simulink model "Tricopter_Controlled"  (R2015a)
settings: Solver=ode3  SolverMode=SingleTasking  StartTime=0.0  StopTime=inf  FixedStep=T_sim  RelTol=1e-3
values from neighbouring files (symbols this model uses):
  A_l_max_x = sqrt( (A_z_max)^2  -  g^2  )    [Run3Copter.m]
  A_l_max_y = g*tand(15)    [Run3Copter.m]
  A_z_max = Max_Thrust*3/m    [Run3Copter.m]
  Alt_0 = input(' Give the initial altitude (m): ')    [Run3Copter.m]
  B_hover_4dof = [-0.192641491537 -0.295051706147 -72.3190840892 -0.00308714144823 24.9504828653 -1.18743631629 9.87469464114e-05 6.48783896558 -0.0529805907426 -0.000387203135788 0.131620058452 2.24065603044 ... (54 elements, 6x9)]    [Effectiv_matrices.mat]
  CG_0 = [0,0,0.02]'    [SetupComplete.m]
  epsilon = 0.01    [Run3Copter.m]
  eta_23 = deg2rad(-1.3)    [Run3Copter.m]
  g = 9.81    [SetupComplete.m]
  h = 0.08    [SetupComplete.m]
  h_M = 0.064    [SetupComplete.m]
  Hover_eta_23 = deg2rad(-1.3)    [Run3Copter.m]
  Hover_throtle_1 = 0.745    [Run3Copter.m]
  Hover_throtle_23 = Hover_throtle_1/cos(Hover_eta_23)    [Run3Copter.m]
  I_BAC_0 = [ Ix,0,Ixz;0,Iy,0;Ixz,0,Iz]    [SetupComplete.m]
  Initial_Omegas = Omega_hover    [Run3Copter.m]
  Initial_Torques = Torque_hover    [Run3Copter.m]
  Ix = 0.103    [SetupComplete.m]
  Iy = 0.147    [SetupComplete.m]
  Iz = 0.237    [SetupComplete.m]
  l = 0.345    [SetupComplete.m]
  l_arm = 0.264    [SetupComplete.m]
  latitude = 52.071118    [Run3Copter.m]
  longitude = -0.627404    [Run3Copter.m]
  m = 3.51    [SetupComplete.m]
  m_0 = 2.61    [SetupComplete.m]
  m_M = 0.300    (= 0.3)    [SetupComplete.m]
  Rotation_sign = [ 1,-1,-1]    [SetupComplete.m]
  T_ctrl = 0.02    [Run3Copter.m]
  T_sim = 0.01    [Run3Copter.m]
  throtle_1 = 0*0.745    (= 0)    [Run3Copter.m]
  throtle_23 = throtle_1/cos(eta_23)    [Run3Copter.m]
  v_i0 = sqrt( 1/3*m*g/(2*rho*pi*R^2)  )    [SetupComplete.m]
undefined symbols (not defined in the file or in its folder): DOWN_0, EAST_0, Newton, NORTH_0, P_0, Q_0, R_0, Raphson, U_0, V_0, W_0
libraries: XXCopter_Control x64, simulink_extras x17, simulink x11, XXCopter x8
(part 1 of 6)
settings Model: ExtModeTrigDuration=5000  Creator=DavidTorres  LastModifiedBy=David
settings SolverCC: AutoInsertRateTranBlk=on
settings DataIOCC: LimitDataPoints=off  SaveOutput=off  SignalLogging=off  DSMLogging=off  VisualizeSimOutput=off  SaveTime=off
settings OptimizationCC: InlineParams=on  UseFloatMulNetSlope=on  UseSpecifiedMinMax=on  InlineInvariantSignals=on  EnhancedBackFolding=on  PassReuseOutputArgsAs=Individual arguments  ZeroExternalMemoryAtStartup=off  ZeroInternalMemoryAtStartup=off  EfficientFloat2IntCast=on  EfficientMapNaN2IntZero=off  OptimizeModelRefInitCode=on  LifeSpan=Inf  MaxStackSize=inf
settings DebuggingCC: WriteAfterWriteMsg=EnableAllAsError  SaveWithParameterizedLinksMsg=none  SignalResolutionControl=TryResolveAllWithWarning  IntegerOverflowMsg=error  ParameterUnderflowMsg=error  ParameterTunabilityLossMsg=error  UniqueDataStoreMsg=error  StrictBusMsg=ErrorOnBusTreatedAsVector  NonBusSignalsTreatedAsBus=error  SFUnexpectedBacktrackingDiag=error  SFInvalidInputDataAccessInChartInitDiag=error  SFNoUnconditionalDefaultTransitionDiag=error  SFTransitionOutsideNaturalParentDiag=error  SFUnconditionalTransitionShadowingDiag=error  SFUndirectedBroadcastEventsDiag=error  SFTransitionActionBeforeConditionDiag=error  IntegerSaturationMsg=error
settings HardwareCC: ProdLargestAtomicInteger=Long  ProdLargestAtomicFloat=Float  ProdIntDivRoundTo=Zero  ProdEndianess=LittleEndian  ProdHWDeviceType=ARM Compatible->ARM 10
settings RTWCC: SystemTargetFile=ert.tlc  GenCodeOnly=on  TemplateMakefile=ert_default_tmf  Description=Embedded Coder  BuildConfiguration=Faster Runs  CheckMdlBeforeBuild=Warning
settings CodeAppCC: IgnoreCustomStorageClasses=off  IgnoreTestpoints=on
settings ERTTargetCC: UtilityFuncGeneration=Shared location  ParMdlRefBuildCompliant=on  CompOptLevelCompliant=on  ConcurrentExecutionCompliant=on  IncludeMdlTerminateFcn=off  ERTFirstTimeCompliant=on  SupportAbsoluteTime=off  SupportNonFinite=off  SupportContinuousTime=off  ParenthesesLevel=Minimum  ModelStepFunctionPrototypeControlCompliant=on  CPPClassGenCompliant=on  ERTCustomFileTemplate=example_file_process.tlc  PreserveIfCondition=on  ConvertIfToSwitch=on

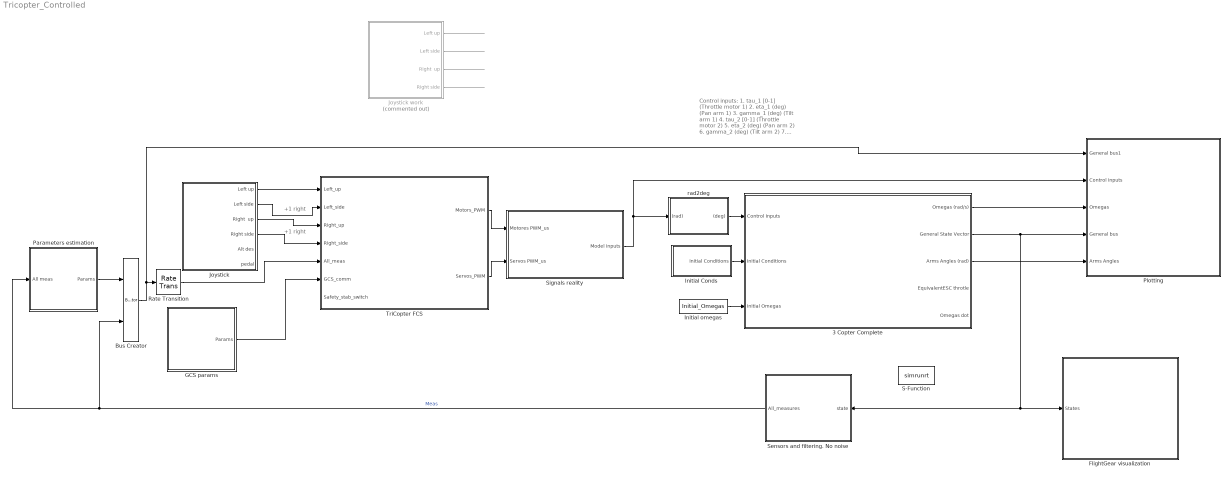
== system Tricopter_Controlled ==
  note: +1 right
  note: Control inputs:
      | 1. tau_1 [0-1] (Throttle motor 1)
      | 2. eta_1 (deg)  (Pan arm 1)
      | 3. gamma_1 (deg)  (Tilt arm 1)
      |
      | 4. tau_2 [0-1] (Throttle motor 2)
      | 5. eta_2 (deg)  (Pan arm 2)
      | 6. gamma_2 (deg)  (Tilt arm 2)
      |
      | 7. tau_3 [0-1] (Throttle motor 3)
      | 8. eta_3 (deg)  (Pan arm  3)
      | 9. gamma_3 (deg)  (Tilt arm 3)
  note: +1 right
  3 Copter Complete : Subsystem
  Bus Creator : BusCreator  Inputs=2
  FlightGear visualization : Subsystem
      mask Display:
      | % disp('{\bf\fontsize{20} Flight Gear}', 'texmode','on');
      | % image('FG F16.jpg')
      | % image(imread('FlightGear_logo.png'))
  GCS params : Subsystem  TreatAsAtomicUnit=on
  Initial Conds : Subsystem  TreatAsAtomicUnit=on
  Initial omegas : Constant  Value=Initial_Omegas
  Joystick : Subsystem
  Joystick work : Subsystem  Commented=on
  Parameters estimation : Subsystem  TreatAsAtomicUnit=on
  Plotting : Subsystem  SystemSampleTime=T_ctrl
  Rate Transition : RateTransition  OutPortSampleTime=T_ctrl
  S-Function : S-Function  FunctionName=simrunrt  Parameters=1
  Sensors and filtering. No noise : Subsystem  Variant=on  VariantControl=No noise  OverrideUsingVariant=No noise
  Signals reality : Subsystem
  TriCopter FCS : Subsystem
  rad2deg : Subsystem  TreatAsAtomicUnit=on
  wires:
  Initial omegas/1 -> 3 Copter Complete/3(Initial Omegas)
  Initial Conds/1(Initial Conditions) -> 3 Copter Complete/2(Initial Conditions)
  3 Copter Complete/1(Omegas (rad/s)) -> Plotting/3(Omegas)
  3 Copter Complete/3(Arms Angles (rad)) -> Plotting/5(Arms Angles)
  rad2deg/1((deg)) -> 3 Copter Complete/1(Control Inputs)
  Sensors and filtering. No noise/1(All_measures) -> Parameters estimation/1(All meas), Bus Creator/2  "Meas"
  3 Copter Complete/2(General State Vector) -> Plotting/4(General bus), Sensors and filtering. No noise/1(state), FlightGear visualization/1(States)
  Bus Creator/1 -> Rate Transition/1, Plotting/1(General bus1)
  Parameters estimation/1(Params) -> Bus Creator/1
  Signals reality/1(Model inputs) -> Plotting/2(Control inputs), rad2deg/1((rad))
  TriCopter FCS/1(Motors_PWM) -> Signals reality/1(Motores PWM_us)
  TriCopter FCS/2(Servos_PWM) -> Signals reality/2(Servos PWM_us)
  GCS params/1(Params) -> TriCopter FCS/6(GCS_comm)
  Joystick/1(Left up) -> TriCopter FCS/1(Left_up)
  Joystick/2(Left side) -> TriCopter FCS/2(Left_side)
  Joystick/3(Right  up) -> TriCopter FCS/3(Right_up)
  Joystick/4(Right side) -> TriCopter FCS/4(Right_side)
  Joystick work/4(Right side) -> ?
  Joystick work/1(Left up) -> ?
  Joystick work/2(Left side) -> ?
  Joystick work/3(Right  up) -> ?
  Rate Transition/1 -> TriCopter FCS/5(All_meas)

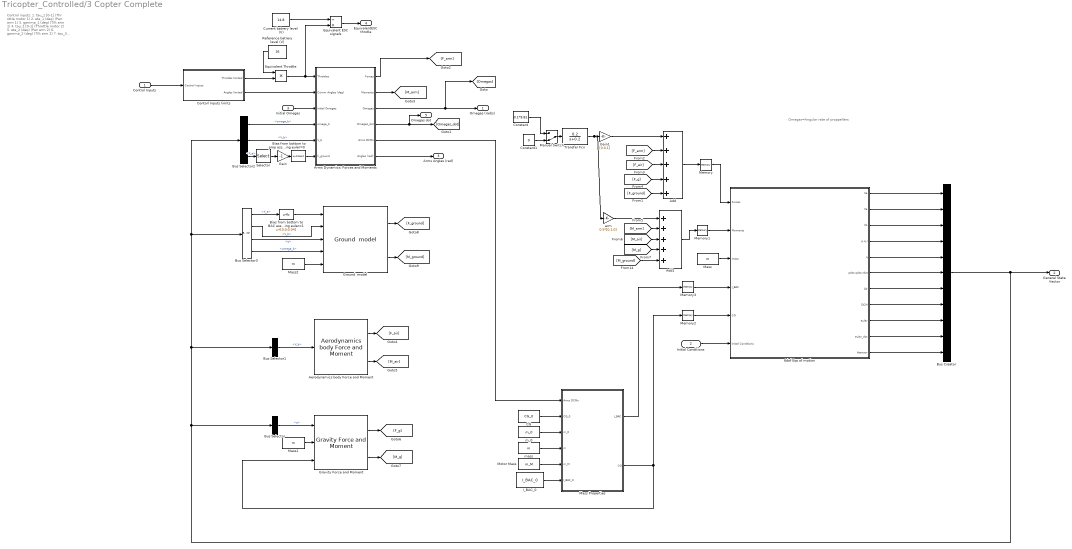
== system Tricopter_Controlled/3 Copter Complete ==
  note: Omegas=Angular rate of proppellers
  note: Control inputs:
      | 1. tau_1 [0-1] (Thr ottle motor 1)
      | 2. eta_1 (deg)  (Pan arm 1)
      | 3. gamma_1 (deg)  (Tilt arm 1)
      |
      | 4. tau_2 [0-1] (Throttle motor 2)
      | 5. eta_2 (deg)  (Pan arm 2)
      | 6. gamma_2 (deg)  (Tilt arm 2)
      |
      | 7. tau_3 [0-1] (Throttle motor 3)
      | 8. eta_3 (deg)  (Pan arm  3)
      | 9. gamma_3 (deg)  (Tilt arm 3)
  Control Inputs : Inport
  Initial Conditions : Inport  Port=2
  Initial Omegas : Inport  Port=3
  6dof Eqs of motion : Subsystem  TreatAsAtomicUnit=on
  Add : Sum  Inputs=+++++
  Add1 : Sum  Inputs=+++++
  Aerodynamics body Force and Moment : XXCopter/Aerodynamics body Force and Moment
  Arms Dynamics: Forces and Moments : Subsystem
  Bias from bottom to BAC assuming euler=1 : Bias  Bias=[0;0;0.04]
  Bias from bottom to prop assuming euler=0 : Bias  Bias=0.04+h
  Bus Creator : BusCreator  Inputs=11
  Bus Selector : BusSelector  OutputSignals=q
  Bus Selector1 : BusSelector  OutputSignals=V_b
  Bus Selector2 : BusSelector  OutputSignals=omega_b,V_b,X_e
  Bus Selector3 : BusSelector  OutputSignals=X_e,V_b,q,omega_b
  CG : Constant  Value=CG_0
  Constant : Constant  Value=0.1*9.81
  Constant1 : Constant  Value=0
  Contorl Inputs limits : Subsystem  TreatAsAtomicUnit=on
  Current batrery level (V) : Constant  Value=14.8
  Equivalent ESC signals : Product  Inputs=/*
  Equivalent Throttle : Product  Inputs=**
  Gain : Gain  Gain=-1
  Gain1 : Gain  Gain=[0,0,1]
  Gravity Force and Moment : XXCopter/Gravity Force and Moment
  Ground  model : XXCopter/Ground  model
  I_BAC_0 : Constant  Value=I_BAC_0
  Manual Switch : ManualSwitch  CurrentSetting=0
  Mass : Constant  Value=m
  Mass Properties : Subsystem  TreatAsAtomicUnit=on
  Mass1 : Constant  Value=m
  Mass2 : Constant  Value=m
  Memory : Memory  X0=[0,0,0]
  Memory1 : Memory  X0=[0,0,0]
  Memory2 : Memory  X0=CG_0
  Memory3 : Memory  X0=I_BAC_0
  Motor Mass : Constant  Value=m_M
  Reference batrery level (V) : Constant  Value=16
  Selector : Selector  InputPortWidth=3  Indices=3
  Transfer Fcn : TransferFcn  Numerator=[0.2]  Denominator=[1 0.2]
  arm : Gain  Gain=0.5*[0,1,0]
  m_0 : Constant  Value=m_0
  mass : Constant  Value=m
  Omegas (rad/s) : Outport
  General State Vector : Outport  Port=2
  Arms Angles (rad) : Outport  Port=3
  EquivalentESC throtle : Outport  Port=4
  Omegas dot : Outport  Port=5
  wires:
  Initial Conditions/1 -> 6dof Eqs of motion/6(Initial Conditions)
  6dof Eqs of motion/3(Vb) -> Bus Creator/3
  6dof Eqs of motion/5(q) -> Bus Creator/5
  6dof Eqs of motion/2(Ve) -> Bus Creator/2
  6dof Eqs of motion/6(pdot,qdot,rdot) -> Bus Creator/6
  6dof Eqs of motion/1(Xe) -> Bus Creator/1
  6dof Eqs of motion/7(Ab) -> Bus Creator/7
  6dof Eqs of motion/8(DCM) -> Bus Creator/8
  6dof Eqs of motion/9(euler) -> Bus Creator/9
  6dof Eqs of motion/10(euler_dot) -> Bus Creator/10
  Bus Selector/1 -> Gravity Force and Moment/1  "<q>"
  Mass/1 -> 6dof Eqs of motion/3(mass)
  Mass Properties/1(I_BAC) -> Memory3/1
  Bus Selector1/1 -> Aerodynamics body Force and Moment/1  "<V_b>"
  Bus Selector2/1 -> Arms Dynamics: Forces and Moments/4(omega_b)  "<omega_b>"
  Bus Selector2/2 -> Arms Dynamics: Forces and Moments/5(V_b)  "<V_b>"
  Mass1/1 -> Gravity Force and Moment/2
  Mass Properties/2(CG) -> Gravity Force and Moment/3, Memory2/1
  Arms Dynamics: Forces and Moments/4(Omegas_dot) -> Omegas dot/1, [Omegas_dot]
  Initial Omegas/1 -> Arms Dynamics: Forces and Moments/3(Initial Omegas)
  Bus Selector2/3 -> Selector/1  "<X_e>"
  Selector/1 -> Gain/1
  Gain/1 -> Bias from bottom to prop assuming euler=0/1
  Add/1 -> Memory/1
  Add1/1 -> Memory1/1
  Arms Dynamics: Forces and Moments/1(Forces) -> [F_arm]
  Arms Dynamics: Forces and Moments/2(Moments) -> [M_arm]
  Aerodynamics body Force and Moment/1 -> [F_air]
  Aerodynamics body Force and Moment/2 -> [M_air]
  Gravity Force and Moment/1 -> [F_g]
  Gravity Force and Moment/2 -> [M_g]
  [F_arm] -> Add/2
  [F_air] -> Add/3
  [F_g] -> Add/4
  6dof Eqs of motion/11(Asensor) -> Bus Creator/11
  Contorl Inputs limits/1(Throtles limited) -> Equivalent Throttle/2
  Contorl Inputs limits/2(Angles limited) -> Arms Dynamics: Forces and Moments/2(Comm Angles (deg))
  Arms Dynamics: Forces and Moments/5(Arms DCMs) -> Mass Properties/1(Arms DCMs)
  CG/1 -> Mass Properties/2(CG_0)
  Motor Mass/1 -> Mass Properties/5(m_M)
  I_BAC_0/1 -> Mass Properties/6(I_BAC_0)
  m_0/1 -> Mass Properties/3(m_0)
  mass/1 -> Mass Properties/4(m)
  Arms Dynamics: Forces and Moments/3(Omegas) -> [Omegas], Omegas (rad/s)/1
  Memory/1 -> 6dof Eqs of motion/1(Forces)
  Memory1/1 -> 6dof Eqs of motion/2(Moments)
  Memory2/1 -> 6dof Eqs of motion/5(CG)
  Memory3/1 -> 6dof Eqs of motion/4(I_BAC)
  Equivalent Throttle/1 -> Equivalent ESC signals/2, Arms Dynamics: Forces and Moments/1(Throttles)
  Reference batrery level (V)/1 -> Equivalent Throttle/1
  Current batrery level (V)/1 -> Equivalent ESC signals/1
  Equivalent ESC signals/1 -> EquivalentESC throtle/1
  6dof Eqs of motion/4(p,q,r) -> Bus Creator/4
  Arms Dynamics: Forces and Moments/6(Angles (rad)) -> Arms Angles (rad)/1
  Control Inputs/1 -> Contorl Inputs limits/1(Control inputs)
  [M_g] -> Add1/4
  [M_air] -> Add1/3
  [M_arm] -> Add1/2
  Transfer Fcn/1 -> arm/1, Gain1/1
  arm/1 -> Add1/1
  Manual Switch/1 -> Transfer Fcn/1
  Constant/1 -> Manual Switch/1
  Constant1/1 -> Manual Switch/2
  Gain1/1 -> Add/1
  Bus Creator/1 -> Bus Selector3/1, Bus Selector2/1, Bus Selector1/1, Bus Selector/1, General State Vector/1
  Ground  model/1 -> [F_ground]
  Ground  model/2 -> [M_ground]
  [F_ground] -> Add/5
  [M_ground] -> Add1/5
  Bus Selector3/1 -> Bias from bottom to BAC assuming euler=1/1  "<X_e>"
  Bus Selector3/3 -> Ground  model/3  "<q>"
  Mass2/1 -> Ground  model/5
  Bus Selector3/2 -> Ground  model/2  "<V_b>"
  Bus Selector3/4 -> Ground  model/4  "<omega_b>"
  Bias from bottom to BAC assuming euler=1/1 -> Ground  model/1
  Bias from bottom to prop assuming euler=0/1 -> Arms Dynamics: Forces and Moments/6(h_ground)

== system Tricopter_Controlled/FlightGear visualization ==
  note: States Dot:
      | 1. DEV North Position
      | 2. DEV East position
      | 3. DEV Altitude
      | 4.DEV  Phi
      | 5. DEV Theta
      | 6. DEV Psi
      | 7. DEV Total velocity
      | 8.DEV alpha in rad
      | 9.DEV  beta in rads
      | 10. DEV P
      | 11. DEV Q
      | 12. DEV R
  note: States:
      | 1. North Position
      | 2. East position
      | 3. Altitude
      | 4. Phi
      | 5. Theta
      | 6. Psi
      | 7. Total velocity
      | 8. alpha in rad
      | 9. beta in rads
      | 10. P
      | 11. Q
      | 12. R
      | 13 POW
  States : Inport
  Bus Selector2 : BusSelector  OutputSignals=X_e,euler
  Demux : Demux  Outputs=3
  Flat Earth to LLA : Subsystem
  Mux : Mux  Inputs=6
  Saturation : Saturate  UpperLimit=1e8  LowerLimit=-1e5  OutDataTypeStr=double
  Send2FG : S-Function  FunctionName=sim2fg  Parameters='localhost',5502
  cast1 : DataTypeConversion  OutDataTypeStr=double  SaturateOnIntegerOverflow=on
  href : Constant  Value=100  VectorParams1D=off
  keep pi/pi : Subsystem
  wires:
  Demux/2 -> Mux/5
  Demux/1 -> Mux/4
  href/1 -> Flat Earth to LLA/2(altitude0)
  Saturation/1 -> Mux/3
  Bus Selector2/1 -> Flat Earth to LLA/1(Xe)  "<X_e>"
  Mux/1 -> cast1/1
  cast1/1 -> Send2FG/1
  keep pi/pi/1(ptp_earth) -> Demux/1
  Demux/3 -> Mux/6
  Flat Earth to LLA/3(altitude h) -> Saturation/1
  Flat Earth to LLA/1(latitude mu) -> Mux/1
  Flat Earth to LLA/2(longitude l) -> Mux/2
  States/1 -> Bus Selector2/1
  Bus Selector2/2 -> keep pi/pi/1(phi theta psi)  "<euler>"

== system Tricopter_Controlled/GCS params ==
  Bus Creator : BusCreator  Inputs=10
  Constant : Constant
  Constant{1,4..8,10} (7 alike) : Constant  Value=0
  FM_source : Constant  Value=0  SampleTime=T_sim
  FM_source1 : Constant  SampleTime=T_sim
  FM_source2 : Constant  Value=2  SampleTime=T_sim
  FM_source3 : Constant  Value=3  SampleTime=T_sim
  Manual Switch : ManualSwitch  CurrentSetting=0
  Manual Switch1 : ManualSwitch  CurrentSetting=0
  Manual Switch2 : ManualSwitch  CurrentSetting=0
  theta_comm : Constant  Value=0  SampleTime=T_sim
  Params : Outport
  wires:
  Bus Creator/1 -> Params/1  "Params"
  Constant/1 -> Bus Creator/3  "Alt_com"
  Constant1/1 -> Bus Creator/1  "X_com"
  Manual Switch2/1 -> Bus Creator/10  "flight_mode_request"
  Constant4/1 -> Bus Creator/2  "Y_com"
  Constant5/1 -> Bus Creator/4  "Vx_yaw_com"
  Constant6/1 -> Bus Creator/5  "Vy_yaw_com"
  Constant7/1 -> Bus Creator/6  "Vz_yaw_com"
  Constant8/1 -> Bus Creator/7  "phi_com_deg"
  theta_comm/1 -> Bus Creator/8  "theta_com_deg"
  Constant10/1 -> Bus Creator/9  "heading_com_deg"
  FM_source/1 -> Manual Switch/1  "flight_mode_request"
  FM_source1/1 -> Manual Switch/2
  Manual Switch/1 -> Manual Switch1/1
  FM_source2/1 -> Manual Switch1/2
  Manual Switch1/1 -> Manual Switch2/1
  FM_source3/1 -> Manual Switch2/2

== system Tricopter_Controlled/Initial Conds ==
  Bus Creator : BusCreator
  Ini Position X_e_0 : Constant  Value=[0;0;-Alt_0]
  Initial Attitude Euler_0 : Constant  Value=[deg2rad(0);deg2rad(0);deg2rad(0)]
  Initial Attitude Rate  Euler_dot_0 : Constant  Value=[deg2rad(0);deg2rad(0);deg2rad(0)]
  Initial Velocity V_e_0 : Constant  Value=[0;0;0]
  Initial Conditions : Outport
  wires:
  Ini Position X_e_0/1 -> Bus Creator/1  "X_e_0"
  Initial Velocity V_e_0/1 -> Bus Creator/2  "V_e_0"
  Initial Attitude Euler_0/1 -> Bus Creator/3  "Euler_0"
  Initial Attitude Rate  Euler_dot_0/1 -> Bus Creator/4  "Euler_dot_0"
  Bus Creator/1 -> Initial Conditions/1

== system Tricopter_Controlled/Joystick ==
  Add2 : Sum
  Aileron : Selector  InputPortWidth=2
  Aileron1 : Selector  InputPortWidth=2
  Gain{1,3,5,8} (4 alike) : Gain
  Gain2 : Gain  Gain=-1
  Gain4 : Gain  Gain=-1
  Gain6 : Gain  Gain=0.1  OutDataTypeStr=double
  Gain7 : Gain  Gain=-1
  Integrator Limited2 : Integrator  LimitOutput=on  UpperSaturationLimit=400  LowerSaturationLimit=-400
  S-Function : S-Function  FunctionName=joyinput  Parameters=joyid,adjustports,forcefeed  mask{joyid=1, adjustports=on, forcefeed=off}
      mask prompts: joyid "Joystick ID:"; adjustports "Adjust ports?"; forcefeed "Enable force"
      mask init:
      | label = 'image(imread(''joystickicon.png'')); port_label(''output'', 1, ''Axes''); port_label(''output'', 2, ''Buttons''); ';
      | porthandles = get_param(gcbh, 'PortHandles');
      | if numel(porthandles.Outport)>2
      |   label = [label 'port_label(''output'', 3, ''Point of View''); '];
      | end
      | if numel(porthandles.Inport)>0  label = [label 'port_label(''input'', 1, ''Force''); '];
      | end
      | set_param(gcbh, 'MaskDisplay', label);
      mask Help: helpview(vrmfunc('FnHelpTopic'), 'vr_joystickinput');
      mask Display: image(imread('joystickicon.png')); port_label('output', 1, 'Axes'); port_label('output', 2, 'Buttons'); port_label('output', 3, 'Point of View');
  Selector1 : Selector  InputPortWidth=5  Indices=1:2
  Selector2 : Selector  InputPortWidth=5  Indices=3
  Selector3 : Selector  InputPortWidth=5  Indices=4:5
  Selector6 : Selector  InputPortWidth=10
  Selector7 : Selector  InputPortWidth=10  Indices=4
  Terminator : Terminator
  elev : Selector  InputPortWidth=2  Indices=2
  elev1 : Selector  InputPortWidth=2  Indices=2
  Left up : Outport
  Left side : Outport  Port=2
  Right  up : Outport  Port=3
  Right side : Outport  Port=4
  Alt des : Outport  Port=5
  pedal : Outport  Port=6
  wires:
  Aileron/1 -> Gain1/1
  Selector1/1 -> Aileron/1, elev/1
  S-Function/1 -> Selector1/1, Selector2/1, Selector3/1
  elev/1 -> Gain2/1
  Gain1/1 -> Left side/1
  Gain2/1 -> Left up/1
  Selector2/1 -> Gain5/1
  Integrator Limited2/1 -> Alt des/1
  S-Function/2 -> Selector7/1, Selector6/1
  Selector6/1 -> Gain7/1
  Selector7/1 -> Gain8/1
  Gain7/1 -> Add2/1
  Gain8/1 -> Add2/2
  Add2/1 -> Gain6/1
  Gain6/1 -> Integrator Limited2/1
  ? -> Terminator/1
  Gain5/1 -> pedal/1
  Aileron1/1 -> Gain3/1
  elev1/1 -> Gain4/1
  Gain3/1 -> Right side/1
  Gain4/1 -> Right  up/1
  Selector3/1 -> Aileron1/1, elev1/1

== system Tricopter_Controlled/Joystick work ==
  Add2 : Sum
  Aileron1 : Selector  InputPortWidth=2
  Gain{1..3,7} (4 alike) : Gain
  Gain4 : Gain  Gain=-1
  Gain6 : Gain  Gain=0.1  OutDataTypeStr=double
  Gain8 : Gain  Gain=-1
  Integrator Limited2 : Integrator  LimitOutput=on  UpperSaturationLimit=400  LowerSaturationLimit=-400
  S-Function : S-Function  FunctionName=joyinput  Parameters=joyid,adjustports,forcefeed  mask{joyid=2, adjustports=on, forcefeed=off}
      mask prompts: joyid "Joystick ID:"; adjustports "Adjust ports?"; forcefeed "Enable force"
      mask init: same as Tricopter_Controlled/Joystick/S-Function
      mask Help: helpview(vrmfunc('FnHelpTopic'), 'vr_joystickinput');
      mask Display: image(imread('joystickicon.png')); port_label('output', 1, 'Axes'); port_label('output', 2, 'Buttons');
  Selector1 : Selector  InputPortWidth=4  Indices=1:2
  Selector2 : Selector  InputPortWidth=4  Indices=4
  Selector6 : Selector  InputPortWidth=12
  Selector7 : Selector  InputPortWidth=12  Indices=2
  Terminator : Terminator
  elev1 : Selector  InputPortWidth=2  Indices=2
  Left up : Outport
  Left side : Outport  Port=2
  Right  up : Outport  Port=3
  Right side : Outport  Port=4
  wires:
  Selector2/1 -> Gain1/1
  S-Function/1 -> Selector1/1, Selector2/1
  Integrator Limited2/1 -> Gain2/1
  Gain1/1 -> Left side/1
  Gain2/1 -> Left up/1
  S-Function/2 -> Selector7/1, Selector6/1
  Selector6/1 -> Gain7/1
  Selector7/1 -> Gain8/1
  Gain7/1 -> Add2/1
  Gain8/1 -> Add2/2
  Add2/1 -> Gain6/1
  Gain6/1 -> Integrator Limited2/1
  ? -> Terminator/1
  Aileron1/1 -> Gain3/1
  elev1/1 -> Gain4/1
  Gain3/1 -> Right side/1
  Gain4/1 -> Right  up/1
  Selector1/1 -> Aileron1/1, elev1/1

== system Tricopter_Controlled/Parameters estimation ==
  note: This is T_Fb->Fe
  All meas : Inport
  Bus Creator : BusCreator  Inputs=7
  Bus Selector : BusSelector  OutputSignals=A_accel meas,Euler meas (rad),V_e_meas
  DCM1 : Subsystem  TreatAsAtomicUnit=on
  GPS_sat : Constant  Value=5
  MATLAB Function : MATLAB Function  TreatAsAtomicUnit=on
  Matrix Multiply1 : Product  Multiplication=Matrix(*)
  Matrix Multiply2 : Product  Multiplication=Matrix(*)
  Permute Dimensions : PermuteDimensions
  Selector1 : Selector  InputPortWidth=3  Indices=3
  Selector7 : Selector  InputPortWidth=3  Indices=[3 2 1]
  Sum : Sum  Inputs=++|
  g : Constant  Value=[0;0;g]
  gps_vdop : Constant  Value=1.5
  p_dop : Constant  Value=1.5
  Params : Outport
  wires:
  All meas/1 -> Bus Selector/1
  Bus Selector/2 -> Selector1/1, Selector7/1  "<Euler meas (rad)>"
  DCM1/1(DCM) -> Permute Dimensions/1, Bus Creator/2  "DCM"
  Selector7/1 -> DCM1/1(Euler)
  Bus Creator/1 -> Params/1  "Params"
  Selector1/1 -> MATLAB Function/1(yaw)
  MATLAB Function/1(T_yaw) -> Matrix Multiply2/1, Bus Creator/3  "T_Fe-Fyaw"
  Matrix Multiply2/1 -> Bus Creator/4  "V_yaw"
  Bus Selector/3 -> Matrix Multiply2/2  "<V_e_meas>"
  Permute Dimensions/1 -> Matrix Multiply1/1
  g/1 -> Matrix Multiply1/2
  Matrix Multiply1/1 -> Sum/2
  Bus Selector/1 -> Sum/1  "<A_accel meas>"
  Sum/1 -> Bus Creator/1  "a_meas"
  p_dop/1 -> Bus Creator/5  "gps_pdop"
  GPS_sat/1 -> Bus Creator/7  "gps_sat"
  gps_vdop/1 -> Bus Creator/6  "gps_vdop"

== system Tricopter_Controlled/Plotting ==
  General bus1 : Inport
  Control inputs : Inport  Port=2
  Omegas : Inport  Port=3
  General bus : Inport  Port=4
  Arms Angles : Inport  Port=5
  3Copt anim : Subsystem  Commented=on
  Actual ang arm 1 : simulink_extras/Transformations/Radians to Degrees
  Actual ang arm2 : simulink_extras/Transformations/Radians to Degrees
  Actual ang arm3 : simulink_extras/Transformations/Radians to Degrees
  Arms dynamics : Scope  NumInputPorts=3
      settings: ShowLegends=on  TimeRange=50  YMin=-100~-150~-200  YMax=200~150~200  SaveName=ScopeData2
  Bus Selector : BusSelector  OutputSignals=euler,omega_b,X_e,V_e,DCM
  Bus Selector1 : BusSelector  OutputSignals=Angles Arm 1,Angles Arm 2,Angles Arm 3
  Bus Selector2 : BusSelector  OutputSignals=Meas.Euler meas (rad),Meas.omega_b meas (rad/s),Meas.Pos meas (m),Meas.V_e_meas
  Comm ang arm1 : simulink_extras/Transformations/Radians to Degrees
  Comm ang arm2 : simulink_extras/Transformations/Radians to Degrees
  Comm ang arm3 : simulink_extras/Transformations/Radians to Degrees
  Demux : Demux  Outputs=3
  Demux1 : Demux  Outputs=3
  Euler omega_b : Scope  NumInputPorts=2
      settings: ShowLegends=on  TimeRange=50  YMin=-35~-10  YMax=5~7.5
  MEas Position Velocity : Scope  NumInputPorts=2
      settings: ShowLegends=on  TimeRange=100  YMin=-4~-2.5  YMax=1~1.5  SaveName=ScopeData6
  Meas Euler omega_b : Scope  NumInputPorts=2
      settings: ShowLegends=on  TimeRange=100  YMin=-2.5~-5  YMax=17.5~17.5  SaveName=ScopeData5
  Mux : Mux  Inputs=3
  Mux1 : Mux  Inputs=2
  Mux2 : Mux  Inputs=2
  Mux3 : Mux  Inputs=2
  Mux4 : Mux  Inputs=3
  Position Velocity : Scope  NumInputPorts=2
      settings: ShowLegends=on  TimeRange=50  YMin=-1.5~-1.5  YMax=0.25~1.5  SaveName=ScopeData8
  Radians to Degrees{,1..3} (4 alike) : simulink_extras/Transformations/Radians to Degrees
  Rotors states : Scope  NumInputPorts=2
      settings: ShowLegends=on  TimeRange=100  YMin=0~0  YMax=0.6~800
  angles arm 2 : Selector  InputPortWidth=9  Indices=[5,6]
  angles arm 3 : Selector  InputPortWidth=9  Indices=[8,9]
  "angles arm2 " : Selector  InputPortWidth=9  Indices=[2,3]
  throtles : Selector  InputPortWidth=9  Indices=[1,4,7]
  wires:
  General bus/1 -> Bus Selector/1
  Bus Selector/1 -> Radians to Degrees/1  "<euler>"
  Omegas/1 -> Rotors states/2  "Omegas"
  Arms Angles/1 -> Bus Selector1/1
  Mux3/1 -> 3Copt anim/5(In5), Arms dynamics/3
  Mux2/1 -> 3Copt anim/4(In4), Arms dynamics/2
  Mux1/1 -> 3Copt anim/3(In3), Arms dynamics/1
  Bus Selector/3 -> 3Copt anim/1(In1), Position Velocity/1  "<X_e>"
  Demux/3 -> Mux/3  "psi(deg)"
  Demux/1 -> Mux/1  "phi(deg)"
  Demux/2 -> Mux/2  "theta(deg)"
  Mux/1 -> Euler omega_b/1
  Bus Selector/2 -> Radians to Degrees1/1  "<omega_b>"
  Control inputs/1 -> "angles arm2 "/1, angles arm 3/1, angles arm 2/1, throtles/1
  Bus Selector1/1 -> Actual ang arm 1/1  "<Angles Arm 1>"
  "angles arm2 "/1 -> Comm ang arm1/1
  Bus Selector1/2 -> Actual ang arm2/1  "<Angles Arm 2>"
  angles arm 2/1 -> Comm ang arm2/1
  Bus Selector1/3 -> Actual ang arm3/1  "<Angles Arm 3>"
  angles arm 3/1 -> Comm ang arm3/1
  throtles/1 -> Rotors states/1
  Radians to Degrees/1 -> Demux/1
  Comm ang arm1/1 -> Mux1/2
  Actual ang arm3/1 -> Mux3/1
  Actual ang arm2/1 -> Mux2/1
  Actual ang arm 1/1 -> Mux1/1
  Comm ang arm2/1 -> Mux2/2
  Comm ang arm3/1 -> Mux3/2
  Bus Selector/4 -> Position Velocity/2  "<V_e>"
  Radians to Degrees1/1 -> Euler omega_b/2  "omega_b (deg/s)"
  Bus Selector2/1 -> Radians to Degrees2/1  "<Euler meas (rad)>"
  Bus Selector2/3 -> MEas Position Velocity/1  "<Pos meas (m)>"
  Demux1/3 -> Mux4/3  "psi(deg)"
  Demux1/1 -> Mux4/1  "phi(deg)"
  Demux1/2 -> Mux4/2  "theta(deg)"
  Mux4/1 -> Meas Euler omega_b/1
  Bus Selector2/2 -> Radians to Degrees3/1  "<omega_b meas (rad/s)>"
  Radians to Degrees2/1 -> Demux1/1
  Bus Selector2/4 -> MEas Position Velocity/2  "<V_e_meas>"
  Radians to Degrees3/1 -> Meas Euler omega_b/2  "omega_b (deg/s)"
  General bus1/1 -> Bus Selector2/1
  Bus Selector/5 -> 3Copt anim/2(In2)  "<DCM>"

== system Tricopter_Controlled/Sensors and filtering. No noise ==
  state : Inport
  Sensors and filtering. No noise : Subsystem  VariantControl=No noise
  Sensors and filtering. Noise : Subsystem  VariantControl=Noise
  All_measures : Outport

== system Tricopter_Controlled/Signals reality ==
  Motores PWM_us : Inport
  Servos PWM_us : Inport  Port=2
  Memory : Memory  X0=[throtle_1,throtle_23,throtle_23]'  InheritSampleTime=on
  Memory1 : Memory  X0=[0,0,eta_23,0,-eta_23,0]'  InheritSampleTime=on
  Mux : Mux  Inputs=[1,2,1,2,1,2]
  PWM resolution : Subsystem  TreatAsAtomicUnit=on
  PWM resolution1 : Subsystem  TreatAsAtomicUnit=on
  PWM2signal1 : XXCopter_Control/PWM2signal  c=1800  a=1200  d=1  b=0
  Rate Transition1 : RateTransition  OutPortSampleTime=T_ctrl
  Rate Transition2 : RateTransition  OutPortSampleTime=T_ctrl
  Re-Build Signals servos : Subsystem  TreatAsAtomicUnit=on
  Selector : Selector  InputPortWidth=3
  Selector1 : Selector  InputPortWidth=3  Indices=2
  Selector2 : Selector  InputPortWidth=3  Indices=3
  Selector3 : Selector  InputPortWidth=6  Indices=[1,2]
  Selector4 : Selector  InputPortWidth=6  Indices=[3,4]
  Selector5 : Selector  InputPortWidth=6  Indices=[5,6]
  Model inputs : Outport
  wires:
  Motores PWM_us/1 -> PWM resolution/1(PWM_us in)
  Memory/1 -> Rate Transition1/1
  PWM resolution/1(PWM_us out) -> PWM2signal1/1
  Servos PWM_us/1 -> PWM resolution1/1(PWM_us in)
  Re-Build Signals servos/1(signals out) -> Memory1/1
  PWM resolution1/1(PWM_us out) -> Re-Build Signals servos/1(PWM_us servos in)
  Memory1/1 -> Rate Transition2/1
  Mux/1 -> Model inputs/1
  Rate Transition1/1 -> Selector2/1, Selector1/1, Selector/1
  Selector/1 -> Mux/1
  Selector2/1 -> Mux/5
  Selector1/1 -> Mux/3
  Rate Transition2/1 -> Selector5/1, Selector4/1, Selector3/1
  Selector3/1 -> Mux/2
  Selector4/1 -> Mux/4
  Selector5/1 -> Mux/6
  PWM2signal1/1 -> Memory/1

== system Tricopter_Controlled/TriCopter FCS ==
  Left_up : Inport
  Left_side : Inport  Port=2
  Right_up : Inport  Port=3
  Right_side : Inport  Port=4
  All_meas : Inport  Port=5
  GCS_comm : Inport  Port=6
  Safety_stab_switch : Inport  Port=7
  Interface out : Subsystem
  Simulink to px4 input : Subsystem  TreatAsAtomicUnit=on
  TriCopter FCS : Subsystem  TreatAsAtomicUnit=on
  Motors_PWM : Outport
  Servos_PWM : Outport  Port=2
  wires:
  TriCopter FCS/1(pwm1) -> Interface out/1(In1)
  TriCopter FCS/2(pwm2) -> Interface out/2(In2)
  TriCopter FCS/3(pwm3) -> Interface out/3(In3)
  TriCopter FCS/4(pwm4) -> Interface out/4(In4)
  TriCopter FCS/5(pwm5) -> Interface out/5(In5)
  TriCopter FCS/6(pwm6) -> Interface out/6(In6)
  TriCopter FCS/7(pwm7) -> Interface out/7(In7)
  TriCopter FCS/8(pwm8) -> Interface out/8(In8)
  Interface out/1(Out1) -> Motors_PWM/1
  Interface out/2(Out2) -> Servos_PWM/1
  Left_up/1 -> Simulink to px4 input/1(Left_up)
  Left_side/1 -> Simulink to px4 input/2(Left_side)
  Right_up/1 -> Simulink to px4 input/3(Right_up)
  Right_side/1 -> Simulink to px4 input/4(Right_side)
  GCS_comm/1 -> Simulink to px4 input/6(GCS_comm)
  Safety_stab_switch/1 -> Simulink to px4 input/7(Safety_stab_switch)
  All_meas/1 -> Simulink to px4 input/5(All_meas)
  Simulink to px4 input/10(gyro_y) -> TriCopter FCS/10(gyro_y)
  Simulink to px4 input/11(gyro_z) -> TriCopter FCS/11(gyro_z)
  Simulink to px4 input/12(acc_x) -> TriCopter FCS/12(acc_x)
  Simulink to px4 input/13(acc_y) -> TriCopter FCS/13(acc_y)
  Simulink to px4 input/14(acc_z) -> TriCopter FCS/14(acc_z)
  Simulink to px4 input/15(mag_x) -> TriCopter FCS/15(mag_x)
  Simulink to px4 input/16(mag_y) -> TriCopter FCS/16(mag_y)
  Simulink to px4 input/17(mag_z) -> TriCopter FCS/17(mag_z)
  Simulink to px4 input/18(baro_alt) -> TriCopter FCS/18(baro_alt)
  Simulink to px4 input/19(gps_sat) -> TriCopter FCS/19(gps_sat)
  Simulink to px4 input/20(gps_lat) -> TriCopter FCS/20(gps_lat)
  Simulink to px4 input/21(gps_lon) -> TriCopter FCS/21(gps_lon)
  Simulink to px4 input/22(gps_alt) -> TriCopter FCS/22(gps_alt)
  Simulink to px4 input/23(gps_vel) -> TriCopter FCS/23(gps_vel)
  Simulink to px4 input/24(gps_vel_n) -> TriCopter FCS/24(gps_vel_n)
  Simulink to px4 input/25(gps_vel_e) -> TriCopter FCS/25(gps_vel_e)
  Simulink to px4 input/26(gps_vel_d) -> TriCopter FCS/26(gps_vel_d)
  Simulink to px4 input/27(sonar_dist) -> TriCopter FCS/27(sonar_dist)
  Simulink to px4 input/28(flow_x) -> TriCopter FCS/28(flow_x)
  Simulink to px4 input/29(flow_y) -> TriCopter FCS/29(flow_y)
  Simulink to px4 input/30(rate_roll) -> TriCopter FCS/30(rate_roll)
  Simulink to px4 input/31(rate_pitch) -> TriCopter FCS/31(rate_pitch)
  Simulink to px4 input/32(rate_yaw) -> TriCopter FCS/32(rate_yaw)
  Simulink to px4 input/33(att_roll) -> TriCopter FCS/33(att_roll)
  Simulink to px4 input/34(att_pitch) -> TriCopter FCS/34(att_pitch)
  Simulink to px4 input/35(att_yaw) -> TriCopter FCS/35(att_yaw)
  Simulink to px4 input/36(q0) -> TriCopter FCS/36(q0)
  Simulink to px4 input/37(q1) -> TriCopter FCS/37(q1)
  Simulink to px4 input/38(q2) -> TriCopter FCS/38(q2)
  Simulink to px4 input/39(q3) -> TriCopter FCS/39(q3)
  Simulink to px4 input/40(runtime) -> TriCopter FCS/40(runtime)
  Simulink to px4 input/41(Lo_pos_x) -> TriCopter FCS/41(Lo_pos_x)
  Simulink to px4 input/42(Lo_pos_y) -> TriCopter FCS/42(Lo_pos_y)
  Simulink to px4 input/43(Lo_pos_z) -> TriCopter FCS/43(Lo_pos_z)
  Simulink to px4 input/44(Lo_vex) -> TriCopter FCS/44(Lo_vex)
  Simulink to px4 input/45(Lo_vey) -> TriCopter FCS/45(Lo_vey)
  Simulink to px4 input/46(Lo_vez) -> TriCopter FCS/46(Lo_vez)
  Simulink to px4 input/47(Lo_yaw) -> TriCopter FCS/47(Lo_yaw)
  Simulink to px4 input/48(gps_pdop) -> TriCopter FCS/48(gps_pdop)
  Simulink to px4 input/49(gps_vdop) -> TriCopter FCS/49(gps_vdop)
  Simulink to px4 input/50(bat_volts) -> TriCopter FCS/50(bat_volts)
  Simulink to px4 input/51(X_comm) -> TriCopter FCS/51(X_comm)
  Simulink to px4 input/52(Y_comm) -> TriCopter FCS/52(Y_comm)
  Simulink to px4 input/53(Alt_comm) -> TriCopter FCS/53(Alt_comm)
  Simulink to px4 input/54(Vx_yaw_comm) -> TriCopter FCS/54(Vx_yaw_comm)
  Simulink to px4 input/55(Vy_yaw_comm) -> TriCopter FCS/55(Vy_yaw_comm)
  Simulink to px4 input/56(Vz_yaw_comm) -> TriCopter FCS/56(Vz_yaw_comm)
  Simulink to px4 input/57(phi_comm) -> TriCopter FCS/57(phi_comm)
  Simulink to px4 input/58(theta_comm) -> TriCopter FCS/58(theta_comm)
  Simulink to px4 input/59(head_comm) -> TriCopter FCS/59(head_comm)
  Simulink to px4 input/60(flight_mode_request) -> TriCopter FCS/60(flight_mode_request)
  Simulink to px4 input/1(ch1) -> TriCopter FCS/1(ch1)
  Simulink to px4 input/2(ch2) -> TriCopter FCS/2(ch2)
  Simulink to px4 input/3(ch3) -> TriCopter FCS/3(ch3)
  Simulink to px4 input/4(ch4) -> TriCopter FCS/4(ch4)
  Simulink to px4 input/5(ch5) -> TriCopter FCS/5(ch5)
  Simulink to px4 input/6(ch6) -> TriCopter FCS/6(ch6)
  Simulink to px4 input/7(ch7) -> TriCopter FCS/7(ch7)
  Simulink to px4 input/8(ch8) -> TriCopter FCS/8(ch8)
  Simulink to px4 input/9(gyro_x) -> TriCopter FCS/9(gyro_x)
  TriCopter FCS/16(debug2) -> Interface out/9(In9)

== system Tricopter_Controlled/rad2deg ==
  (rad) : Inport
  Demux : Demux  Outputs=6
  Demux1 : Demux  Outputs=3
  Mux : Mux  Inputs=9
  Radians to Degrees : simulink_extras/Transformations/Radians to Degrees
  Throttles : Selector  InputPortWidth=9  Indices=[1,4,7]
  "angles " : Selector  InputPortWidth=9  Indices=[2,3,5,6,8,9]
  (deg) : Outport
  wires:
  (rad)/1 -> Throttles/1, "angles "/1
  Throttles/1 -> Demux1/1
  "angles "/1 -> Radians to Degrees/1
  Mux/1 -> (deg)/1
  Radians to Degrees/1 -> Demux/1
  Demux1/1 -> Mux/1
  Demux/1 -> Mux/2
  Demux/2 -> Mux/3
  Demux1/2 -> Mux/4
  Demux/3 -> Mux/5
  Demux/4 -> Mux/6
  Demux1/3 -> Mux/7
  Demux/5 -> Mux/8
  Demux/6 -> Mux/9

== system Tricopter_Controlled/3 Copter Complete/6dof Eqs of motion ==
  note: This is T_Fb->Fe
  note: In rads!
  Forces : Inport
  Moments : Inport  Port=2
  mass : Inport  Port=3
  I_BAC : Inport  Port=4
  CG : Inport  Port=5
  Initial Conditions : Inport  Port=6
  Bus Selector : BusSelector  OutputSignals=X_e_0,V_e_0,Euler_0,Euler_dot_0
  DCM1 : Subsystem  TreatAsAtomicUnit=on
  Eccelerometer meas : MATLAB Function  TreatAsAtomicUnit=on
  Normalize 4D vector : XXCopter/Normalize 4D vector
  Position Eqs : MATLAB Function  TreatAsAtomicUnit=on
  Rotational eqs : MATLAB Function  TreatAsAtomicUnit=on
  SVFI_to_SVFb : MATLAB Function  TreatAsAtomicUnit=on  SystemSampleTime=T_sim
  SV_F_b_to_SV_FI : MATLAB Function  TreatAsAtomicUnit=on
  Selector7 : Selector  InputPortWidth=3  Indices=[3 2 1]
  "p,q,r " : Integrator  InitialConditionSource=external  InitialCondition=[P_0,Q_0,R_0]
  q_dot : Subsystem  TreatAsAtomicUnit=on
  quaternion : Integrator  InitialConditionSource=external  InitialCondition=[P_0,Q_0,R_0]
  ub,vb,wb : Integrator  InitialConditionSource=external  InitialCondition=[U_0,V_0,W_0]
  xe,ye,ze : Integrator  InitialConditionSource=external  InitialCondition=[NORTH_0,EAST_0,-DOWN_0]
  Xe : Outport
  Ve : Outport  Port=2
  Vb : Outport  Port=3
  p,q,r : Outport  Port=4
  q : Outport  Port=5
  pdot,qdot,rdot : Outport  Port=6
  Ab : Outport  Port=7
  DCM : Outport  Port=8
  euler : Outport  Port=9
  euler_dot : Outport  Port=10
  Asensor : Outport  Port=11
  wires:
  I_BAC/1 -> Rotational eqs/3(I_BAC)
  mass/1 -> Position Eqs/5(m)
  Forces/1 -> Position Eqs/4(Forces)
  xe,ye,ze/1 -> Xe/1  "X_e"
  ub,vb,wb/1 -> Vb/1, Eccelerometer meas/1(Vb), Position Eqs/1(Vb), SV_F_b_to_SV_FI/1(V_b)  "V_b"
  SV_F_b_to_SV_FI/1(V_e) -> Ve/1, xe,ye,ze/1  "V_e"
  [omega] -> Position Eqs/2(omega)
  [omega_dot] -> Position Eqs/3(omega_dot)
  Position Eqs/1(A_b) -> Eccelerometer meas/4(Ab), Ab/1, ub,vb,wb/1  "A_b"
  CG/1 -> Position Eqs/6(CG)
  Initial Conditions/1 -> Bus Selector/1
  Bus Selector/1 -> SVFI_to_SVFb/1(X_e)  "<X_e_0>"
  Bus Selector/2 -> SVFI_to_SVFb/2(V_e)  "<V_e_0>"
  Bus Selector/3 -> SVFI_to_SVFb/3(Euler_Ang)  "<Euler_0>"
  Bus Selector/4 -> SVFI_to_SVFb/4(Euler_Ang_Dot)  "<Euler_dot_0>"
  SVFI_to_SVFb/2(V_b) -> ub,vb,wb/2
  SVFI_to_SVFb/1(X_e_out) -> xe,ye,ze/2
  SVFI_to_SVFb/3(omega_b) -> "p,q,r "/2
  Rotational eqs/1(omega_dot) -> pdot,qdot,rdot/1, [omega_dot], "p,q,r "/1
  "p,q,r "/1 -> q_dot/1(omega_b), [omega], p,q,r/1, Rotational eqs/1(omega_b)  "omega_b"
  q_dot/1(q_dot) -> quaternion/1, SV_F_b_to_SV_FI/2(q_dot)
  SVFI_to_SVFb/4(q) -> quaternion/2
  quaternion/1 -> Normalize 4D vector/1, q_dot/2(q)  "q"
  DCM1/1(DCM) -> DCM/1  "DCM"
  SV_F_b_to_SV_FI/2(euler) -> Selector7/1, euler/1  "euler"
  SV_F_b_to_SV_FI/3(euler_dot) -> euler_dot/1  "euler_dot"
  Moments/1 -> Rotational eqs/2(Moments)
  Normalize 4D vector/1 -> q/1, SV_F_b_to_SV_FI/3(q)  "q"
  [omega] -> Eccelerometer meas/2(omega)
  [omega_dot] -> Eccelerometer meas/3(omega_dot)
  Eccelerometer meas/1(A_s) -> Asensor/1
  Selector7/1 -> DCM1/1(Euler)

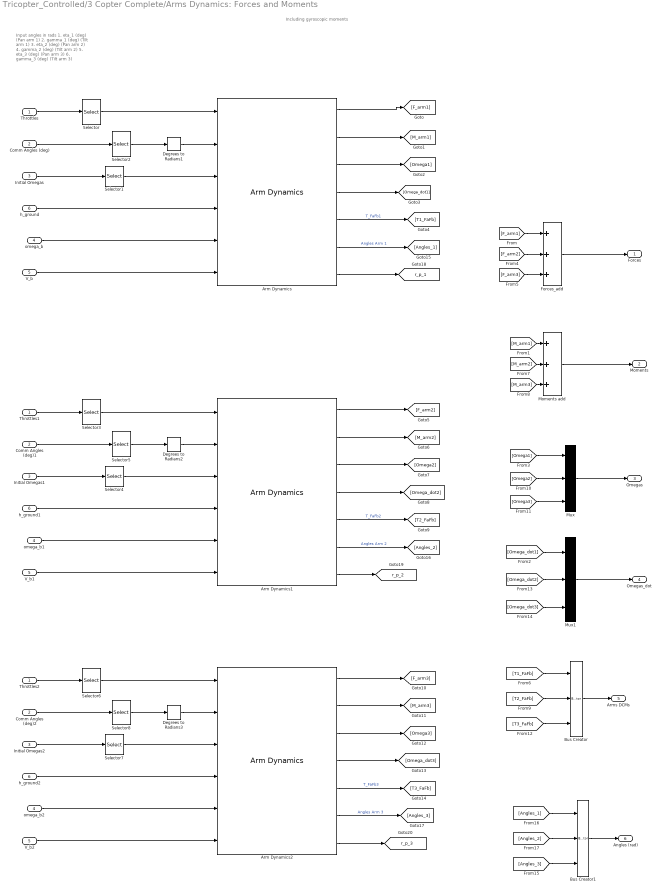
== system Tricopter_Controlled/3 Copter Complete/Arms Dynamics: Forces and Moments ==
  note: Including gyroscopic moments
  note: Input angles in rads
      |
      | 1. eta_1 (deg)  (Pan arm 1)
      | 2. gamma_1 (deg)  (Tilt arm 1)
      |
      | 3. eta_2 (deg)  (Pan arm 2)
      | 4. gamma_2 (deg)  (Tilt arm 2)
      |
      | 5. eta_3 (deg)  (Pan arm  3)
      | 6. gamma_3 (deg)  (Tilt arm 3)
  Throttles : Inport
  Comm Angles (deg) : Inport  Port=2
  Initial Omegas : Inport  Port=3
  omega_b : Inport  Port=4
  V_b : Inport  Port=5
  h_ground : Inport  Port=6
  Arm Dynamics : XXCopter/Arm Dynamics  Rot_sign=Rotation_sign(1)  tau=Tau_motors  arm_hub_pos=l*[1;0;0]  Arm_axis=[l_arm;0;0]  arm_num=1  eta_dir=[1;0;0]  gamma_dir=[0;1;0]  J_T=J_T  J_FA=J_FA  h=h  Torq_ini=Initial_Torques(1)  Omega_ini=Initial_Omegas(1)  init_eta=0  init_gamma=0  omega_n=70  xi=0.72  c=0
  Arm Dynamics1 : XXCopter/Arm Dynamics  Rot_sign=Rotation_sign(2)  tau=Tau_motors  arm_hub_pos=l*[-1/2;sqrt(3)/2;0]  Arm_axis=[0;l_arm;0]  arm_num=2  eta_dir=[0;1;0]  gamma_dir=[1;0;0]  J_T=J_T  J_FA=J_FA  h=h  Torq_ini=Initial_Torques(2)  Omega_ini=Initial_Omegas(2)  init_eta=eta_23  init_gamma=0  omega_n=70  xi=0.72  c=0
  Arm Dynamics2 : XXCopter/Arm Dynamics  Rot_sign=Rotation_sign(3)  tau=Tau_motors  arm_hub_pos=l*[-1/2;-sqrt(3)/2;0]  Arm_axis=[0;-l_arm;0]  arm_num=3  eta_dir=[0;1;0]  gamma_dir=[1;0;0]  J_T=J_T  J_FA=J_FA  h=h  Torq_ini=Initial_Torques(3)  Omega_ini=Initial_Omegas(3)  init_eta=-eta_23  init_gamma=0  omega_n=70  xi=0.72  c=0
  Bus Creator : BusCreator  Inputs=3
  Bus Creator1 : BusCreator  Inputs=3
  Comm Angles (deg)1 : InportShadow  Port=2
  Comm Angles (deg)2 : InportShadow  Port=2
  Degrees to Radians1 : simulink_extras/Transformations/Degrees to Radians
  Degrees to Radians2 : simulink_extras/Transformations/Degrees to Radians
  Degrees to Radians3 : simulink_extras/Transformations/Degrees to Radians
  Forces_add : Sum  Inputs=+++
  Initial Omegas1 : InportShadow  Port=3
  Initial Omegas2 : InportShadow  Port=3
  Moments add : Sum  Inputs=+++
  Mux : Mux  Inputs=3
  Mux1 : Mux  Inputs=3
  Selector : Selector  InputPortWidth=3  Indices=[1]
  Selector1 : Selector  InputPortWidth=3  Indices=[1]
  Selector2 : Selector  InputPortWidth=6  Indices=[1,2]
  Selector3 : Selector  InputPortWidth=3  Indices=2
  Selector4 : Selector  InputPortWidth=3  Indices=2
  Selector5 : Selector  InputPortWidth=6  Indices=[3,4]
  Selector6 : Selector  InputPortWidth=3  Indices=3
  Selector7 : Selector  InputPortWidth=3  Indices=3
  Selector8 : Selector  InputPortWidth=6  Indices=[5,6]
  Throttles1 : InportShadow
  Throttles2 : InportShadow
  V_b1 : InportShadow  Port=5
  V_b2 : InportShadow  Port=5
  h_ground1 : InportShadow  Port=6
  h_ground2 : InportShadow  Port=6
  omega_b1 : InportShadow  Port=4
  omega_b2 : InportShadow  Port=4
  Forces : Outport
  Moments : Outport  Port=2
  Omegas : Outport  Port=3
  Omegas_dot : Outport  Port=4
  Arms DCMs : Outport  Port=5
  Angles (rad) : Outport  Port=6
  tag scope: r_p_1=global, r_p_2=global, r_p_3=global
  wires:
  Selector1/1 -> Arm Dynamics/3
  Throttles/1 -> Selector/1
  Initial Omegas/1 -> Selector1/1
  Selector/1 -> Arm Dynamics/1
  V_b/1 -> Arm Dynamics/6
  Forces_add/1 -> Forces/1
  Moments add/1 -> Moments/1
  Mux/1 -> Omegas/1
  Mux1/1 -> Omegas_dot/1
  h_ground/1 -> Arm Dynamics/4
  Arm Dynamics/1 -> [F_arm1]
  Arm Dynamics/2 -> [M_arm1]
  Arm Dynamics/3 -> [Omega1]
  Arm Dynamics/4 -> [Omega_dot1]
  [F_arm1] -> Forces_add/1
  [M_arm1] -> Moments add/1
  [Omega_dot1] -> Mux1/1
  [Omega1] -> Mux/1
  omega_b/1 -> Arm Dynamics/5
  [F_arm2] -> Forces_add/2
  [F_arm3] -> Forces_add/3
  [Omega2] -> Mux/2
  [Omega3] -> Mux/3
  [Omega_dot2] -> Mux1/2
  [Omega_dot3] -> Mux1/3
  [M_arm3] -> Moments add/3
  [M_arm2] -> Moments add/2
  Degrees to Radians1/1 -> Arm Dynamics/2
  Comm Angles (deg)/1 -> Selector2/1
  Selector2/1 -> Degrees to Radians1/1
  Arm Dynamics/5 -> [T1_FaFb]  "T_FaFb1"
  Bus Creator/1 -> Arms DCMs/1
  [T1_FaFb] -> Bus Creator/1
  Selector4/1 -> Arm Dynamics1/3
  Throttles1/1 -> Selector3/1
  Initial Omegas1/1 -> Selector4/1
  Selector3/1 -> Arm Dynamics1/1
  V_b1/1 -> Arm Dynamics1/6
  h_ground1/1 -> Arm Dynamics1/4
  Arm Dynamics1/1 -> [F_arm2]
  Arm Dynamics1/2 -> [M_arm2]
  Arm Dynamics1/3 -> [Omega2]
  Arm Dynamics1/4 -> [Omega_dot2]
  omega_b1/1 -> Arm Dynamics1/5
  Degrees to Radians2/1 -> Arm Dynamics1/2
  Comm Angles (deg)1/1 -> Selector5/1
  Selector5/1 -> Degrees to Radians2/1
  Arm Dynamics1/5 -> [T2_FaFb]  "T_FaFb2"
  [T2_FaFb] -> Bus Creator/2
  Selector7/1 -> Arm Dynamics2/3
  Throttles2/1 -> Selector6/1
  Initial Omegas2/1 -> Selector7/1
  Selector6/1 -> Arm Dynamics2/1
  V_b2/1 -> Arm Dynamics2/6
  h_ground2/1 -> Arm Dynamics2/4
  Arm Dynamics2/1 -> [F_arm3]
  Arm Dynamics2/2 -> [M_arm3]
  Arm Dynamics2/3 -> [Omega3]
  Arm Dynamics2/4 -> [Omega_dot3]
  omega_b2/1 -> Arm Dynamics2/5
  Degrees to Radians3/1 -> Arm Dynamics2/2
  Comm Angles (deg)2/1 -> Selector8/1
  Selector8/1 -> Degrees to Radians3/1
  Arm Dynamics2/5 -> [T3_FaFb]  "T_FaFb3"
  [T3_FaFb] -> Bus Creator/3
  Bus Creator1/1 -> Angles (rad)/1
  [Angles_1] -> Bus Creator1/1
  [Angles_2] -> Bus Creator1/2
  [Angles_3] -> Bus Creator1/3
  Arm Dynamics/6 -> [Angles_1]  "Angles Arm 1"
  Arm Dynamics1/6 -> [Angles_2]  "Angles Arm 2"
  Arm Dynamics2/6 -> [Angles_3]  "Angles Arm 3"
  Arm Dynamics/7 -> [r_p_1]
  Arm Dynamics1/7 -> [r_p_2]
  Arm Dynamics2/7 -> [r_p_3]

== system Tricopter_Controlled/3 Copter Complete/Contorl Inputs limits ==
  note: limits in degs
  Control inputs : Inport
  Demux : Demux  Outputs=6
  Mux : Mux  Inputs=6
  Saturation : Saturate  UpperLimit=1  LowerLimit=0
  Throttles : Selector  InputPortWidth=9  Indices=[1,4,7]
  "angles " : Selector  InputPortWidth=9  Indices=[2,3,5,6,8,9]
  eta 1 : Saturate  UpperLimit=165  LowerLimit=-165
  eta 2 : Saturate  UpperLimit=165  LowerLimit=-165
  eta 3 : Saturate  UpperLimit=165  LowerLimit=-165
  gamma 2 : Saturate  UpperLimit=90  LowerLimit=-15
  gamma1 : Saturate  UpperLimit=15  LowerLimit=-90
  gamma3 : Saturate  UpperLimit=15  LowerLimit=-90
  Throtles limited : Outport
  Angles limited : Outport  Port=2
  wires:
  Control inputs/1 -> Throttles/1, "angles "/1
  Throttles/1 -> Saturation/1
  "angles "/1 -> Demux/1
  Demux/1 -> eta 1/1
  Demux/2 -> gamma1/1
  Demux/3 -> eta 2/1
  Demux/4 -> gamma 2/1
  Demux/5 -> eta 3/1
  Demux/6 -> gamma3/1
  eta 1/1 -> Mux/1
  gamma1/1 -> Mux/2
  eta 2/1 -> Mux/3
  gamma 2/1 -> Mux/4
  eta 3/1 -> Mux/5
  gamma3/1 -> Mux/6
  Mux/1 -> Angles limited/1
  Saturation/1 -> Throtles limited/1

== system Tricopter_Controlled/3 Copter Complete/Mass Properties ==
  Arms DCMs : Inport
  CG_0 : Inport  Port=2
  m_0 : Inport  Port=3
  m : Inport  Port=4
  m_M : Inport  Port=5
  I_BAC_0 : Inport  Port=6
  Arm Inertia : MATLAB Function  TreatAsAtomicUnit=on
  Bus Selector : BusSelector  OutputSignals=T_FaFb1,T_FaFb2,T_FaFb3
  CG position : Sum
  Divide : Product  Inputs=*/
  Divide1 : Product  Inputs=**
  Divide2 : Product  Inputs=/*
  Divide3 : Product  Inputs=**
  Motors Pos sum : Sum  Inputs=+++
  Total I_BAC : Sum
  I_BAC : Outport
  CG : Outport  Port=2
  wires:
  Arms DCMs/1 -> Bus Selector/1
  Bus Selector/3 -> Arm Inertia/3(T3_FAFb)  "<T_FaFb3>"
  Bus Selector/2 -> Arm Inertia/2(T2_FAFb)  "<T_FaFb2>"
  Bus Selector/1 -> Arm Inertia/1(T1_FAFb)  "<T_FaFb1>"
  Total I_BAC/1 -> I_BAC/1
  m_0/1 -> Divide/1
  m/1 -> Divide/2, Divide2/1
  CG_0/1 -> Divide1/1
  Divide/1 -> Divide1/2
  m_M/1 -> Divide2/2
  CG position/1 -> CG/1
  Divide1/1 -> CG position/1
  Motors Pos sum/1 -> Divide3/1
  Divide2/1 -> Divide3/2
  Divide3/1 -> CG position/2
  Arm Inertia/3(r2_M) -> Motors Pos sum/2
  Arm Inertia/4(r3_M) -> Motors Pos sum/1
  Arm Inertia/1(I_M) -> Total I_BAC/2
  I_BAC_0/1 -> Total I_BAC/1
  Arm Inertia/2(r1_M) -> Motors Pos sum/3

== system Tricopter_Controlled/FlightGear visualization/Flat Earth to LLA ==
  note: Flat Earth to LLA
  Xe : Inport
  altitude0 : Inport  Port=2
  Add : Sum
  Demux1 : Demux  Outputs=3
  Demux2 : Demux  Outputs=2
  Mux : Mux  Inputs=2
  Mux1 : Mux  Inputs=3
  Selector : Selector  InputPortWidth=3  Indices=3
  Unary Minus1 : UnaryMinus
  deg2rad : Gain  Gain=pi/180  SaturateOnIntegerOverflow=on  OutDataTypeStr=Inherit: Same as input  ParamDataTypeStr=Inherit: Same as input
  ne to lat/long : Subsystem  AncestorBlock=navlibrary/ne to lat//long
  latitude mu : Outport
  longitude l : Outport  Port=2
  altitude h : Outport  Port=3
  wires:
  Demux2/1 -> latitude mu/1  "latitude"
  Demux2/2 -> longitude l/1
  Xe/1 -> Demux1/1, Selector/1
  deg2rad/1 -> Demux2/1
  ne to lat/long/1(lat_deg) -> Mux/1
  ne to lat/long/2(long_deg) -> Mux/2
  Mux/1 -> deg2rad/1
  Selector/1 -> Unary Minus1/1
  Add/1 -> altitude h/1
  altitude0/1 -> Add/2
  Mux1/1 -> ne to lat/long/1(Xe)
  Demux1/1 -> Mux1/1
  Demux1/2 -> Mux1/2
  Demux1/3 -> Mux1/3
  Unary Minus1/1 -> Add/1

== system Tricopter_Controlled/FlightGear visualization/keep pi//pi ==
  phi theta psi : Inport
  Constant : Constant  Value=180
  Constant2 : Constant  Value=360
  Gain : Gain  Gain=360
  Math Function2 : Math  Operator=rem  SaturateOnIntegerOverflow=on
  Product : Product  Inputs=*/  RndMeth=Zero
  Rounding Function : Rounding  Operator=fix
  Sum2 : Sum  Inputs=|-+
  deg2rad1 : Gain  Gain=pi/180  SaturateOnIntegerOverflow=on  OutDataTypeStr=Inherit: Same as input  ParamDataTypeStr=Inherit: Same as input
  rad2deg : Gain  Gain=180/pi  SaturateOnIntegerOverflow=on  OutDataTypeStr=Inherit: Same as input  ParamDataTypeStr=Inherit: Same as input
  ptp_earth : Outport
  wires:
  phi theta psi/1 -> rad2deg/1
  Constant/1 -> Product/2
  Product/1 -> Rounding Function/1
  Rounding Function/1 -> Gain/1
  Gain/1 -> Sum2/1
  rad2deg/1 -> Math Function2/1
  Constant2/1 -> Math Function2/2
  Math Function2/1 -> Product/1, Sum2/2
  Sum2/1 -> deg2rad1/1
  deg2rad1/1 -> ptp_earth/1

== system Tricopter_Controlled/Parameters estimation/DCM1 ==
  Euler : Inport  PortDimensions=3
  Fcn11 : Fcn  Expr=u(5)*u(4)
  Fcn12 : Fcn  Expr=u(5)*u(1)
  Fcn13 : Fcn  Expr=-u(2)
  Fcn21 : Fcn  Expr=u(3)*u(2)*u(4) - u(6)*u(1)
  Fcn22 : Fcn  Expr=u(3)*u(2)*u(1) + u(6)*u(4)
  Fcn23 : Fcn  Expr=u(3)*u(5)
  Fcn31 : Fcn  Expr=u(6)*u(2)*u(4) + u(3)*u(1)
  Fcn32 : Fcn  Expr=u(6)*u(2)*u(1) - u(3)*u(4)
  Fcn33 : Fcn  Expr=u(6)*u(5)
  Mux : Mux  Inputs=2
  Mux1 : Mux  Inputs=9
  Reshape : Reshape  OutputDimensionality=Customize  OutputDimensions=[3,3]
  sincos : Trigonometry  Operator=sincos
  DCM : Outport  PortDimensions=[3,3]
  wires:
  Fcn33/1 -> Mux1/9
  Fcn32/1 -> Mux1/8
  Fcn23/1 -> Mux1/6
  Fcn22/1 -> Mux1/5
  Fcn31/1 -> Mux1/7
  Fcn21/1 -> Mux1/4
  Fcn13/1 -> Mux1/3
  Fcn12/1 -> Mux1/2
  Fcn11/1 -> Mux1/1
  Mux/1 -> Fcn22/1, Fcn23/1, Fcn31/1, Fcn33/1, Fcn32/1, Fcn21/1, Fcn13/1, Fcn12/1, Fcn11/1
  sincos/2 -> Mux/2
  sincos/1 -> Mux/1
  Reshape/1 -> DCM/1
  Euler/1 -> sincos/1
  Mux1/1 -> Reshape/1

== system Tricopter_Controlled/Plotting/3Copt anim ==
  In1 : Inport
  In2 : Inport  Port=2
  In3 : Inport  Port=3
  In4 : Inport  Port=4
  In5 : Inport  Port=5
  Degrees to Radians : simulink_extras/Transformations/Degrees to Radians
  Degrees to Radians1 : simulink_extras/Transformations/Degrees to Radians
  Degrees to Radians2 : simulink_extras/Transformations/Degrees to Radians
  Level-2 MATLAB S-Function : M-S-Function  FunctionName=Simulation_3_copter
  wires:
  [r_p_3] -> Level-2 MATLAB S-Function/5
  [r_p_2] -> Level-2 MATLAB S-Function/4
  [r_p_1] -> Level-2 MATLAB S-Function/3
  In2/1 -> Level-2 MATLAB S-Function/2
  Degrees to Radians/1 -> Level-2 MATLAB S-Function/6
  Degrees to Radians1/1 -> Level-2 MATLAB S-Function/7
  Degrees to Radians2/1 -> Level-2 MATLAB S-Function/8
  In3/1 -> Degrees to Radians/1
  In1/1 -> Level-2 MATLAB S-Function/1
  In4/1 -> Degrees to Radians1/1
  In5/1 -> Degrees to Radians2/1
